simulink model "Kinematic_Model_Delta_Psi_Control"  (R2016a)
settings: Solver=ode45  SolverMode=SingleTasking  StartTime=0.0  StopTime=50  FixedStep=0.0001  RelTol=1e-3
values from neighbouring files (symbols this model uses):
  l = 0.3 * scale    (= 1.5)    [play_me_first.m]
  lr = l / 2    (= 0.75)    [play_me_first.m]
  theta0 = 0    [play_me_first.m]
  v = 3    [play_me_first.m]
  x0 = -1    [play_me_first.m]
  y0 = 3    [play_me_first.m]
libraries: simulink x2
settings Model: Creator=library12  LastModifiedBy=Windows.10
settings DataIOCC: LimitDataPoints=on  SaveFormat=Array  SignalLoggingSaveFormat=ModelDataLogs
settings OptimizationCC: BlockReduction=off  BooleanDataType=off
settings DebuggingCC: SaveWithParameterizedLinksMsg=none  UnderspecifiedInitializationDetection=Classic  MergeDetectMultiDrivingBlocksExec=none  SignalResolutionControl=TryResolveAllWithWarning  MultiTaskDSMMsg=warning  MultiTaskCondExecSysMsg=none  StateNameClashWarn=warning
settings HardwareCC: ProdBitPerPointer=32  ProdLargestAtomicFloat=None  ProdIntDivRoundTo=Undefined  ProdEndianess=Unspecified  ProdWordSize=32  ProdHWDeviceType=32-bit Generic  TargetUnknown=on
settings ModelReferenceCC: PropagateSignalLabelsOutOfModel=off
settings ConfigComp: CovModelRefEnable=Off

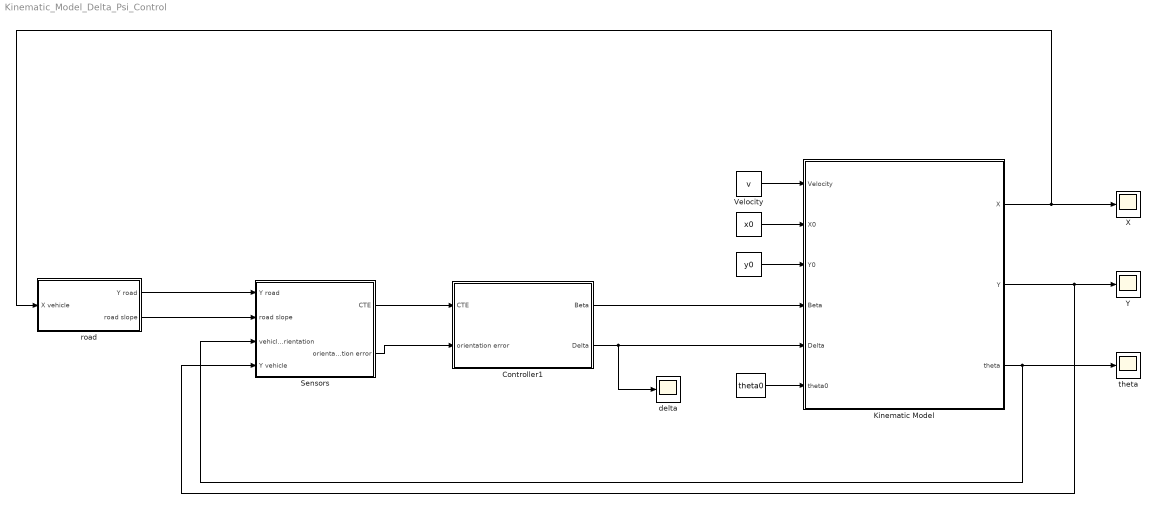
== system Kinematic_Model_Delta_Psi_Control ==
  " " : Constant  Value=x0
  "  " : Constant  Value=y0
  "   " : Constant  Value=theta0
  Controller1 : Subsystem
  Kinematic Model : Subsystem
  Sensors : Subsystem
  "Velocity " : Constant  Value=v
  X : Scope
  Y : Scope
  delta : Scope
  road : Subsystem
  theta : Scope
  wires:
  Controller1/2(Delta) -> Kinematic Model/5(Delta), delta/1
  Controller1/1("Beta ") -> Kinematic Model/4("Beta ")
  Kinematic Model/2(Y) -> Sensors/4(Y vehicle), Y/1
  Kinematic Model/1(X) -> X/1, road/1(X vehicle)
  Kinematic Model/3(theta) -> Sensors/3(vehicle orientation), theta/1
  "Velocity "/1 -> Kinematic Model/1("Velocity ")
  " "/1 -> Kinematic Model/2(X0)
  "  "/1 -> Kinematic Model/3(Y0)
  "   "/1 -> Kinematic Model/6(theta0)
  Sensors/1(CTE) -> Controller1/1(CTE)
  Sensors/2(orientation error) -> Controller1/2(orientation error)
  road/1(Y road) -> Sensors/1(Y road)
  road/2("road slope    ") -> Sensors/2(road slope)

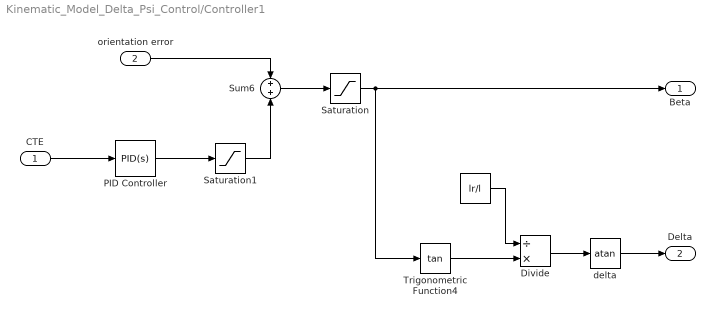
== system Kinematic_Model_Delta_Psi_Control/Controller1 ==
  CTE : Inport
  orientation error : Inport  Port=2
  " " : Constant  Value=lr/l
  Divide : Product  Inputs=/*
  PID Controller : simulink/Continuous/PID Controller  Controller=PID  TimeDomain=Continuous-time  SampleTime=-1  IntegratorMethod=Forward Euler  FilterMethod=Forward Euler  Form=Parallel  UseFilter=on  ControllerParametersSource=internal  P=0.366930822841353  I=0.00322401538585215  D=-0.172843051494264  N=2.12291335792304  InitialConditionSource=internal  InitialConditionForIntegrator=0  InitialConditionForFilter=0  ExternalReset=none  LimitOutput=off  UpperSaturationLimit=pi/2  LowerSaturationLimit=-inf  LinearizeAsGain=on  AntiWindupMode=none  Kb=1  TrackingMode=off  Kt=1  PParamMin=[]  PParamMax=[]  IParamMin=[]  IParamMax=[]  DParamMin=[]  DParamMax=[]  NParamMin=[]  NParamMax=[]  KbParamMin=[]  KbParamMax=[]  KtParamMin=[]  KtParamMax=[]  POutMin=[]  POutMax=[]  IOutMin=[]  IOutMax=[]  DOutMin=[]  DOutMax=[]  NOutMin=[]  NOutMax=[]  KbOutMin=[]  KbOutMax=[]  KtOutMin=[]  KtOutMax=[]  IntegratorOutMin=[]  IntegratorOutMax=[]  FilterOutMin=[]  FilterOutMax=[]  SumOutMin=[]  SumOutMax=[]  SumI1OutMin=[]  SumI1OutMax=[]  SumI2OutMin=[]  SumI2OutMax=[]  SumI3OutMin=[]  SumI3OutMax=[]  SumDOutMin=[]  SumDOutMax=[]  SaturationOutMin=[]  SaturationOutMax=[]  IntegratorContinuousStateAttributes=''  IntegratorStateMustResolveToSignalObject=off  IntegratorRTWStateStorageClass=Auto  FilterContinuousStateAttributes=''  FilterStateMustResolveToSignalObject=off  FilterRTWStateStorageClass=Auto  DifferentiatorICPrevScaledInput=0  DifferentiatorOutMin=[]  DifferentiatorOutMax=[]
  Saturation : Saturate  UpperLimit=pi/6  LowerLimit=-pi/6
  Saturation1 : Saturate  UpperLimit=pi/6  LowerLimit=-pi/6
  Sum6 : Sum
  Trigonometric Function4 : Trigonometry  Operator=tan
  "delta " : Trigonometry  Operator=atan
  "Beta " : Outport
  Delta : Outport  Port=2
  wires:
  Sum6/1 -> Saturation/1
  CTE/1 -> PID Controller/1
  orientation error/1 -> Sum6/1
  PID Controller/1 -> Saturation1/1
  Saturation1/1 -> Sum6/2
  Trigonometric Function4/1 -> Divide/2
  Saturation/1 -> Trigonometric Function4/1, "Beta "/1
  " "/1 -> Divide/1
  Divide/1 -> "delta "/1
  "delta "/1 -> Delta/1

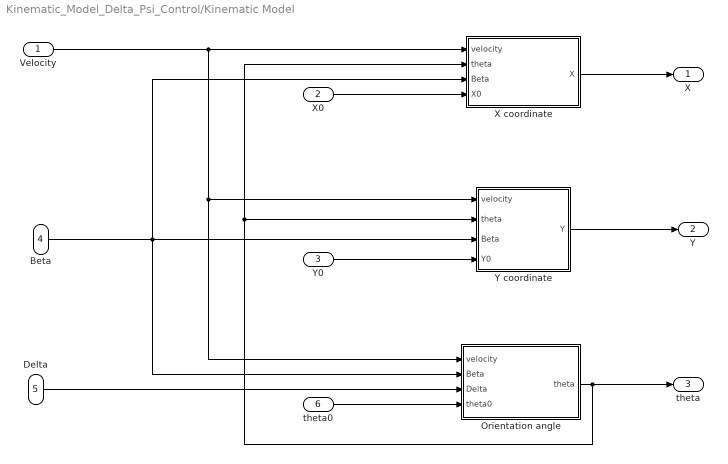
== system Kinematic_Model_Delta_Psi_Control/Kinematic Model ==
  "Velocity " : Inport
  X0 : Inport  Port=2
  Y0 : Inport  Port=3
  "Beta " : Inport  Port=4
  Delta : Inport  Port=5
  theta0 : Inport  Port=6
  Orientation angle : Subsystem
  X coordinate : Subsystem
  Y coordinate : Subsystem
  X : Outport
  Y : Outport  Port=2
  theta : Outport  Port=3
  wires:
  Delta/1 -> Orientation angle/3(Delta)
  "Velocity "/1 -> Orientation angle/1(velocity), Y coordinate/1(velocity), X coordinate/1(velocity)
  theta0/1 -> Orientation angle/4(theta0)
  Y0/1 -> Y coordinate/4(Y0)
  Y coordinate/1(Y) -> Y/1
  X0/1 -> X coordinate/4("X0 ")
  X coordinate/1("X ") -> X/1
  Orientation angle/1(theta) -> X coordinate/2("theta "), Y coordinate/2(theta), theta/1
  "Beta "/1 -> Y coordinate/3(Beta), X coordinate/3(Beta), Orientation angle/2(Beta)

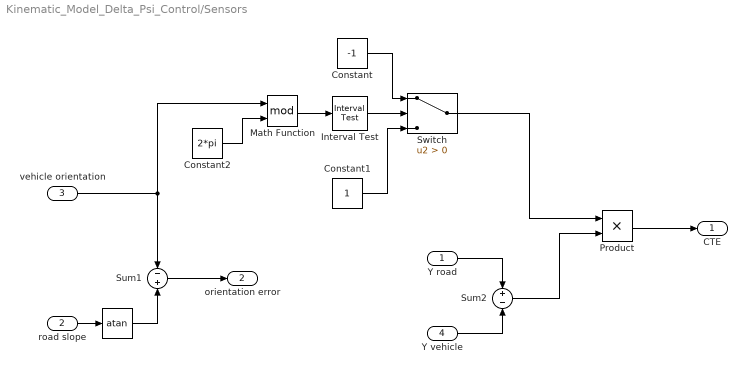
== system Kinematic_Model_Delta_Psi_Control/Sensors ==
  Y road : Inport
  road slope : Inport  Port=2
  vehicle orientation : Inport  Port=3
  Y vehicle : Inport  Port=4
  "                    " : Trigonometry  Operator=atan
  Constant : Constant  Value=-1
  Constant1 : Constant
  Constant2 : Constant  Value=2*pi
  Interval Test : simulink/Logic and Bit Operations/Interval Test  IntervalClosedRight=on  uplimit=3*pi/2  IntervalClosedLeft=on  lowlimit=pi/2  OutDataTypeStr=boolean
  Math Function : Math  Operator=mod  SaturateOnIntegerOverflow=on
  Product : Product
  Sum1 : Sum  Inputs=-+
  Sum2 : Sum  Inputs=+-
  Switch : Switch  Criteria=u2 > Threshold
  CTE : Outport
  orientation error : Outport  Port=2
  wires:
  Sum2/1 -> Product/2
  Sum1/1 -> orientation error/1
  vehicle orientation/1 -> Math Function/1, Sum1/1
  Y vehicle/1 -> Sum2/2
  Constant1/1 -> Switch/3
  Switch/1 -> Product/1
  Math Function/1 -> Interval Test/1
  Constant/1 -> Switch/1
  Interval Test/1 -> Switch/2
  Constant2/1 -> Math Function/2
  "                    "/1 -> Sum1/2
  Product/1 -> CTE/1
  Y road/1 -> Sum2/1
  road slope/1 -> "                    "/1

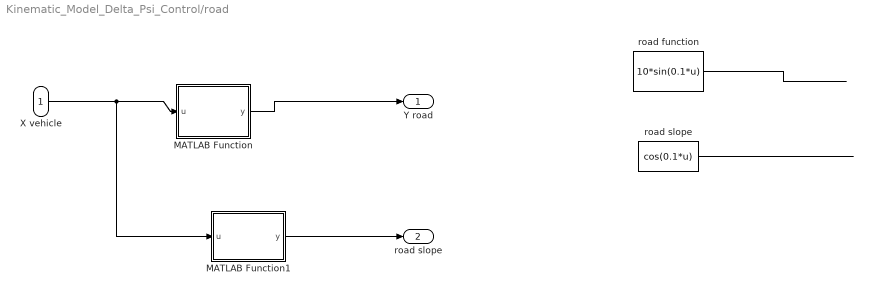
== system Kinematic_Model_Delta_Psi_Control/road ==
  X vehicle : Inport
  MATLAB Function : MATLAB Function  TreatAsAtomicUnit=on
  MATLAB Function1 : MATLAB Function  TreatAsAtomicUnit=on
  road function : Fcn  Expr=10*sin(0.1*u)
  road slope : Fcn  Expr=cos(0.1*u)
  Y road : Outport
  "road slope    " : Outport  Port=2
  wires:
  road slope/1 -> ?
  road function/1 -> ?
  X vehicle/1 -> MATLAB Function1/1(u), MATLAB Function/1(u)
  MATLAB Function/1(y) -> Y road/1
  MATLAB Function1/1(y) -> "road slope    "/1

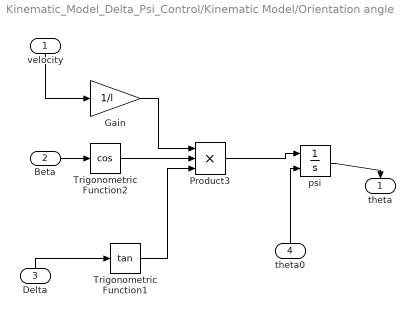
== system Kinematic_Model_Delta_Psi_Control/Kinematic Model/Orientation angle ==
  velocity : Inport
  Beta : Inport  Port=2
  Delta : Inport  Port=3
  theta0 : Inport  Port=4
  Gain : Gain  Gain=1/l
  Product3 : Product  Inputs=3
  Trigonometric Function1 : Trigonometry  Operator=tan
  Trigonometric Function2 : Trigonometry  Operator=cos
  psi : Integrator  InitialConditionSource=external
  theta : Outport
  wires:
  Gain/1 -> Product3/1
  psi/1 -> theta/1
  Trigonometric Function2/1 -> Product3/2
  Trigonometric Function1/1 -> Product3/3
  Product3/1 -> psi/1
  velocity/1 -> Gain/1
  Delta/1 -> Trigonometric Function1/1
  Beta/1 -> Trigonometric Function2/1
  theta0/1 -> psi/2

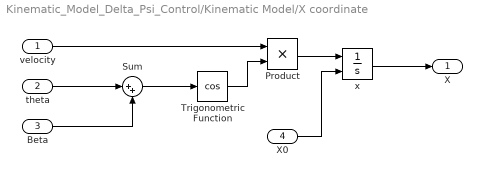
== system Kinematic_Model_Delta_Psi_Control/Kinematic Model/X coordinate ==
  velocity : Inport
  "theta " : Inport  Port=2
  Beta : Inport  Port=3
  "X0 " : Inport  Port=4
  Product : Product
  Sum : Sum  Inputs=|++
  Trigonometric Function : Trigonometry  Operator=cos
  x : Integrator  InitialConditionSource=external
  "X " : Outport
  wires:
  velocity/1 -> Product/1
  "theta "/1 -> Sum/1
  Product/1 -> x/1
  Trigonometric Function/1 -> Product/2
  x/1 -> "X "/1
  Beta/1 -> Sum/2
  Sum/1 -> Trigonometric Function/1
  "X0 "/1 -> x/2

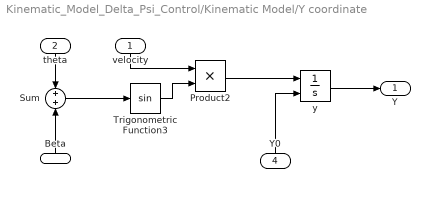
== system Kinematic_Model_Delta_Psi_Control/Kinematic Model/Y coordinate ==
  velocity : Inport
  theta : Inport  Port=2
  Beta : Inport  Port=3
  Y0 : Inport  Port=4
  Product2 : Product
  Sum : Sum
  Trigonometric Function3 : Trigonometry
  "y " : Integrator  InitialConditionSource=external  InitialCondition=1
  Y : Outport
  wires:
  velocity/1 -> Product2/1
  theta/1 -> Sum/1
  Product2/1 -> "y "/1
  Trigonometric Function3/1 -> Product2/2
  "y "/1 -> Y/1
  Beta/1 -> Sum/2
  Sum/1 -> Trigonometric Function3/1
  Y0/1 -> "y "/2

== matlab function Kinematic_Model_Delta_Psi_Control/road/MATLAB Function1 ==
  data: u input; y output
function y = fcn(u)
%#codegen

y = drFcn(u);

== matlab function Kinematic_Model_Delta_Psi_Control/road/MATLAB Function ==
  data: u input; y output
function y = fcn(u)
%#codegen

y = roadFcn(u);
